simulink library "model_lib"  (Simulink 7.8)
settings: Solver=ode45  StartTime=0.0  StopTime=10.0  RelTol=1e-3
settings Model: Creator=mohammad  LastModifiedBy=mai03

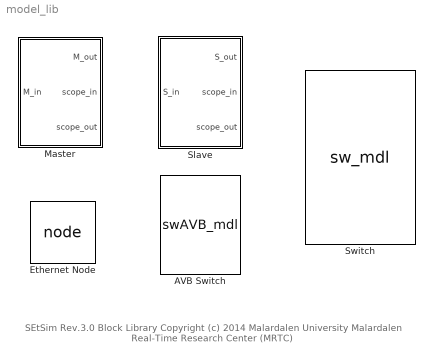
== system model_lib ==
  note: SEtSim Rev.3.0 Block Library
      | Copyright (c) 2014 Malardalen University
      | Malardalen Real-Time Research Center (MRTC)
  AVB Switch : M-S-Function  Priority=1  FunctionName=swAVB_mdl  mask{avb_number=1}
      mask prompts: avb_number "AVB number"
      mask Display:
      | port_label('input',1,'P1')
      | port_label('input',2,'P2')
      | port_label('input',3,'P3')
      | port_label('input',4,'P4')
      | port_label('input',5,'P5')
      | port_label('input',6,'P6')
      | port_label('output',1,'P1')
      | port_label('output',2,'P2')
      | port_label('output',3,'P3')
      | port_label('output',4,'P4')
      | port_label('output',5,'P5')
      | port_label('output',6,'P6')
  Ethernet Node : M-S-Function  FunctionName=node  mask{node_number=1}
      mask prompts: node_number "Node number"
      mask Display:
      | port_label('input',1,'P1')
      | port_label('output',1,'P1')
  Master : Subsystem  Priority=2  mask{master_number=1}
      mask prompts: master_number "Master number"
  Slave : Subsystem  Priority=3  mask{slave_number=1}
      mask prompts: slave_number "Slave number"
  Switch : M-S-Function  Priority=1  FunctionName=sw_mdl  mask{switch_number=1}
      mask prompts: switch_number "Switch number"
      mask Display:
      | port_label('input',1,'M_in')
      | port_label('input',2,'P_SW')
      | port_label('input',3,'C_SW1')
      | port_label('input',4,'C_SW2')
      | port_label('input',5,'C_SW3')
      | port_label('input',6,'C_SW4')
      | port_label('input',7,'P1')
      | port_label('input',8,'P2')
      | port_label('input',9,'P3')
      | port_label('input',10,'P4')
      | port_label('input',11,'P5')
      | port_label('input',12,'P6')
      | port_label('input',13,'P7')
      | port_label('input',14,'P8')
      | port_label('input',15,'P9')
      | port_label('input',16,'P10')
      | port_label('output',1,'M_out')
      | port_label('output',2,'P_SW')
      | port_label('output',3,'C_SW1')
      | port_label('output',4,'C_SW2')
      | port_label('output',5,'C_SW3')
      | port_label('output',6,'C_SW4')
      | port_label('output',7,'P1')
      | port_label('output',8,'P2')
      | port_label('output',9,'P3')
      | port_label('output',10,'P4')
      | port_label('output',11,'P5')
      | port_label('output',12,'P6')
      | port_label('output',13,'P7')
      | port_label('output',14,'P8')
      | port_label('output',15,'P9')
      | port_label('output',16,'P10')

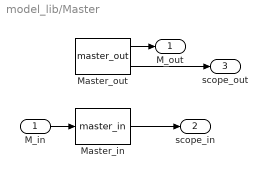
== system model_lib/Master ==
  M_in : Inport
  Master_in : M-S-Function  FunctionName=master_in
  Master_out : M-S-Function  FunctionName=master_out
  M_out : Outport
  scope_in : Outport  Port=2
  scope_out : Outport  Port=3
  wires:
  Master_out/1 -> M_out/1
  M_in/1 -> Master_in/1
  Master_in/1 -> scope_in/1
  Master_out/2 -> scope_out/1

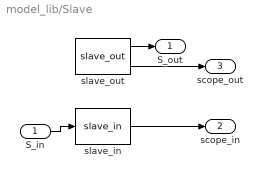
== system model_lib/Slave ==
  S_in : Inport
  slave_in : M-S-Function  FunctionName=slave_in
  slave_out : M-S-Function  FunctionName=slave_out
  S_out : Outport
  scope_in : Outport  Port=2
  scope_out : Outport  Port=3
  wires:
  slave_out/1 -> S_out/1
  S_in/1 -> slave_in/1
  slave_out/2 -> scope_out/1
  slave_in/1 -> scope_in/1
